simulink model "model_LQR"  (R2022b)
settings: Solver=VariableStepAuto  StartTime=0.0  StopTime=30  RelTol=1e-3
values from neighbouring files (symbols this model uses):
  A_INV = [A_P                                        Z1                  Z3                   B_P ... (first row only)    [model_LQR_code.m]
  A_inv = zeros(15,15)    [model_LQR_code.m]
  B_INV = [Z6 ... (first row only)    [model_LQR_code.m]
  B_inv = zeros(15,4)    [model_LQR_code.m]
  C_f = (0.066*C_b)    (= 0.00220630670953)    [model_LQR_code.m]
  C_INV = [C_inv_w ... (first row only)    [model_LQR_code.m]
  C_inv = zeros(2,15)    [model_LQR_code.m]
  D_INV = zeros(3,2)    [model_LQR_code.m]
  D_inv = zeros(2,4)    [model_LQR_code.m]
  f_b = 50    [model_LQR_code.m]
  G3 = -pinv(G2)    [model_LQR_code.m]
  G33 = -pinv(G22)    [model_LQR_code.m]
  Kic = R_f/ti    (= 1.587)    [model_LQR_code.m]
  Kiv = R_f/tiv    (= 0.1587)    [model_LQR_code.m]
  Kpc = L_f/ti    [model_LQR_code.m]
  Kpv = C_f*wm    [model_LQR_code.m]
  L_f = V_dc/(24*f_sw*delta_IL_max)    [model_LQR_code.m]
  L_g = 1*L_f    [model_LQR_code.m]
  mp = 0.03*50*2*pi/(S_b)    (= 1.88495559215e-06)    [model_LQR_code.m]
  nq = 1*V_m/(S_b)    [model_LQR_code.m]
  R_d = 0.2    [model_LQR_code.m]
  R_f = 0.005*Z_b    (= 0.0004761)    [model_LQR_code.m]
  R_g = 0.005*Z_b    (= 0.0004761)    [model_LQR_code.m]
  S_b = 5e6    (= 5000000)    [model_LQR_code.m]
  T_s = 100e-6    (= 0.0001)    [model_LQR_code.m]
  V_dc = 3*V_m    [model_LQR_code.m]
  V_m = sqrt(2/3)*V_b    [model_LQR_code.m]
  w_b = f_b*2*pi    (= 314.159265359)    [model_LQR_code.m]
  w_c = 0.1*w_b    (= 31.4159265359)    [model_LQR_code.m]
undefined symbols (not defined in the file or in its folder): K, K1
libraries: slpidlib x8, spsabctodq0Lib x6, spsThreePhaseSeriesRLCBranchLib x4, spsPowerdq0InstantaneousLib x3, spsThreePhaseVIMeasurementLib x3, spsdq0toabcLib x3, spsGroundLib x2, spsDCVoltageSourceLib x1, spsPLL3phLib x1, spsPWMGenerator2LevelLib x1, spsPower3phPhasorLib x1, spsThreePhaseProgrammableVoltageSourceLib x1
(part 2 of 2)

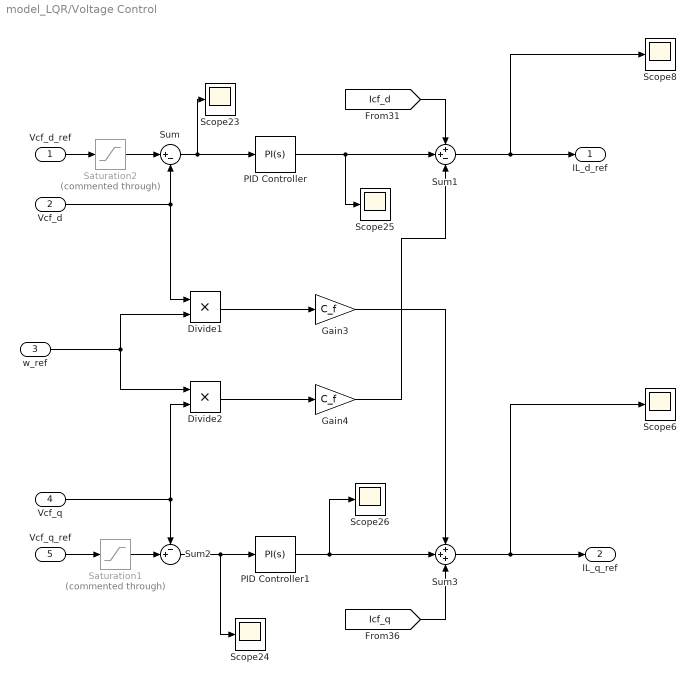
== system model_LQR/Voltage Control ==
  Vcf_d_ref : Inport
  Vcf_d : Inport  Port=2
  w_ref : Inport  Port=3
  Vcf_q : Inport  Port=4
  Vcf_q_ref : Inport  Port=5
  Divide1 : Product  Inputs=**
  Divide2 : Product  Inputs=**
  Gain3 : Gain  Gain=C_f
  Gain4 : Gain  Gain=C_f
  PID Controller : slpidlib/PID Controller  Controller=PI  Form=Parallel  TimeDomain=Continuous-time  UseExternalTs=off  SampleTime=-1  IntegratorMethod=Forward Euler  FilterMethod=Forward Euler  ControllerParametersSource=internal  P=Kpv  I=Kiv  UseKiTs=off  D=0  N=100  UseFilter=on  TunerSelectOption=Transfer Function Based (PID Tuner App)  InitialConditionSource=internal  InitialConditionForIntegrator=0  InitialConditionForFilter=0  DifferentiatorICPrevScaledInput=0  ExternalReset=none  TrackingMode=off  Kt=1  LimitOutput=off  SatLimitsSource=internal  UpperSaturationLimit=75  LowerSaturationLimit=-20  LinearizeAsGain=on  AntiWindupMode=none  Kb=1  LimitIntegrator=off  UpperIntegratorSaturationLimit=inf  LowerIntegratorSaturationLimit=-inf  POutMin=[]  POutMax=[]  IOutMin=[]  IOutMax=[]  DOutMin=[]  DOutMax=[]  NOutMin=[]  NOutMax=[]  SumOutMin=[]  SumOutMax=[]  SaturationOutMin=[]  SaturationOutMax=[]  PParamMin=[]  PParamMax=[]  IParamMin=[]  IParamMax=[]  DParamMin=[]  DParamMax=[]  NParamMin=[]  NParamMax=[]  KbParamMin=[]  KbParamMax=[]  KtParamMin=[]  KtParamMax=[]  KbOutMin=[]  KbOutMax=[]  KtOutMin=[]  KtOutMax=[]  IntegratorOutMin=[]  IntegratorOutMax=[]  FilterOutMin=[]  FilterOutMax=[]  SumI1OutMin=[]  SumI1OutMax=[]  SumI2OutMin=[]  SumI2OutMax=[]  SumI3OutMin=[]  SumI3OutMax=[]  SumI4OutMin=[]  SumI4OutMax=[]  SumDOutMin=[]  SumDOutMax=[]  DifferentiatorOutMin=[]  DifferentiatorOutMax=[]  FilterDiffOutCoefMin=[]  FilterDiffOutCoefMax=[]  ReciprocalOutMin=[]  ReciprocalOutMax=[]  SumDenOutMin=[]  SumDenOutMax=[]  SumNumOutMin=[]  SumNumOutMax=[]  DivideOutMin=[]  DivideOutMax=[]  UdiffTsProdOutMin=[]  UdiffTsProdOutMax=[]  NTsProdOutMin=[]  NTsProdOutMax=[]  UintegralTsProdOutMin=[]  UintegralTsProdOutMax=[]  UngainTsProdOutMin=[]  UngainTsProdOutMax=[]  ClampingZeroOutDataTypeStr=Inherit: Inherit via back propagation  ClampingZeroOutMin=[]  ClampingZeroOutMax=[]  FilterDenConstantOutDataTypeStr=Inherit: Inherit via back propagation  FilterDenConstantOutMin=[]  FilterDenConstantOutMax=[]  PCopyOutDataTypeStr=Inherit: Inherit via back propagation  PCopyOutMin=[]  PCopyOutMax=[]  NCopyOutDataTypeStr=Inherit: Inherit via back propagation  NCopyOutMin=[]  NCopyOutMax=[]  IntegratorContinuousStateAttributes=''  IntegratorStateMustResolveToSignalObject=off  IntegratorRTWStateStorageClass=Auto  FilterContinuousStateAttributes=''  FilterStateMustResolveToSignalObject=off  FilterRTWStateStorageClass=Auto  ParallelPVariant=InternalParameters  IdealPVariant=Disabled  IVariant=InternalParameters  DVariant=Disabled  IntegratorVariant=Continuous  SatVariant=Disabled  AWVariant=Passthrough  PCopyVariant=Disabled  TRVariant=Disabled  FdbkBlocksVariant=Forward  IdealPFdbkVariant=Disabled  SatFdbkVariant=Disabled  DerivativeFilterVariant=Disabled  NVariant=Disabled  NCopyVariant=Disabled_SignalSpec  FilterICVariant=Disabled  IntegratorICVariant=InternalICs  ExternalResetVariant=Disabled  TRSumVariant=Passthrough  SumFdbkVariant=Disabled  SumVariant=Sum_PI  TsampFilterVariant=InternalTs  TsampNgainVariant=Passthrough  TsampIntegralVariant=Passthrough  ExternalSaturationOutDataTypeStr=Inherit: Same as second input
  PID Controller1 : slpidlib/PID Controller  Controller=PI  Form=Parallel  TimeDomain=Continuous-time  UseExternalTs=off  SampleTime=-1  IntegratorMethod=Forward Euler  FilterMethod=Forward Euler  ControllerParametersSource=internal  P=Kpv  I=Kiv  UseKiTs=off  D=0  N=100  UseFilter=on  TunerSelectOption=Transfer Function Based (PID Tuner App)  InitialConditionSource=internal  InitialConditionForIntegrator=0  InitialConditionForFilter=0  DifferentiatorICPrevScaledInput=0  ExternalReset=none  TrackingMode=off  Kt=1  LimitOutput=off  SatLimitsSource=internal  UpperSaturationLimit=250  LowerSaturationLimit=-250  LinearizeAsGain=on  AntiWindupMode=none  Kb=1  LimitIntegrator=off  UpperIntegratorSaturationLimit=inf  LowerIntegratorSaturationLimit=-inf  POutMin=[]  POutMax=[]  IOutMin=[]  IOutMax=[]  DOutMin=[]  DOutMax=[]  NOutMin=[]  NOutMax=[]  SumOutMin=[]  SumOutMax=[]  SaturationOutMin=[]  SaturationOutMax=[]  PParamMin=[]  PParamMax=[]  IParamMin=[]  IParamMax=[]  DParamMin=[]  DParamMax=[]  NParamMin=[]  NParamMax=[]  KbParamMin=[]  KbParamMax=[]  KtParamMin=[]  KtParamMax=[]  KbOutMin=[]  KbOutMax=[]  KtOutMin=[]  KtOutMax=[]  IntegratorOutMin=[]  IntegratorOutMax=[]  FilterOutMin=[]  FilterOutMax=[]  SumI1OutMin=[]  SumI1OutMax=[]  SumI2OutMin=[]  SumI2OutMax=[]  SumI3OutMin=[]  SumI3OutMax=[]  SumI4OutMin=[]  SumI4OutMax=[]  SumDOutMin=[]  SumDOutMax=[]  DifferentiatorOutMin=[]  DifferentiatorOutMax=[]  FilterDiffOutCoefMin=[]  FilterDiffOutCoefMax=[]  ReciprocalOutMin=[]  ReciprocalOutMax=[]  SumDenOutMin=[]  SumDenOutMax=[]  SumNumOutMin=[]  SumNumOutMax=[]  DivideOutMin=[]  DivideOutMax=[]  UdiffTsProdOutMin=[]  UdiffTsProdOutMax=[]  NTsProdOutMin=[]  NTsProdOutMax=[]  UintegralTsProdOutMin=[]  UintegralTsProdOutMax=[]  UngainTsProdOutMin=[]  UngainTsProdOutMax=[]  ClampingZeroOutDataTypeStr=Inherit: Inherit via back propagation  ClampingZeroOutMin=[]  ClampingZeroOutMax=[]  FilterDenConstantOutDataTypeStr=Inherit: Inherit via back propagation  FilterDenConstantOutMin=[]  FilterDenConstantOutMax=[]  PCopyOutDataTypeStr=Inherit: Inherit via back propagation  PCopyOutMin=[]  PCopyOutMax=[]  NCopyOutDataTypeStr=Inherit: Inherit via back propagation  NCopyOutMin=[]  NCopyOutMax=[]  IntegratorContinuousStateAttributes=''  IntegratorStateMustResolveToSignalObject=off  IntegratorRTWStateStorageClass=Auto  FilterContinuousStateAttributes=''  FilterStateMustResolveToSignalObject=off  FilterRTWStateStorageClass=Auto  ParallelPVariant=InternalParameters  IdealPVariant=Disabled  IVariant=InternalParameters  DVariant=Disabled  IntegratorVariant=Continuous  SatVariant=Disabled  AWVariant=Passthrough  PCopyVariant=Disabled  TRVariant=Disabled  FdbkBlocksVariant=Forward  IdealPFdbkVariant=Disabled  SatFdbkVariant=Disabled  DerivativeFilterVariant=Disabled  NVariant=Disabled  NCopyVariant=Disabled_SignalSpec  FilterICVariant=Disabled  IntegratorICVariant=InternalICs  ExternalResetVariant=Disabled  TRSumVariant=Passthrough  SumFdbkVariant=Disabled  SumVariant=Sum_PI  TsampFilterVariant=InternalTs  TsampNgainVariant=Passthrough  TsampIntegralVariant=Passthrough  ExternalSaturationOutDataTypeStr=Inherit: Same as second input
  Saturation1 : Saturate  Commented=through  UpperLimit=30  LowerLimit=-10
  Saturation2 : Saturate  Commented=through  UpperLimit=1.4*V_m  LowerLimit=0.75*V_m
  Scope{6,8,23..26} (6 alike) : Scope
  Sum : Sum  Inputs=|+-
  Sum1 : Sum  Inputs=++-
  Sum2 : Sum  Inputs=-+|
  Sum3 : Sum  Inputs=+++
  IL_d_ref : Outport
  IL_q_ref : Outport  Port=2
  wires:
  Sum/1 -> Scope23/1, PID Controller/1
  PID Controller/1 -> Scope25/1, Sum1/2
  PID Controller1/1 -> Scope26/1, Sum3/2
  [Icf_q] -> Sum3/3
  Gain3/1 -> Sum3/1
  Sum2/1 -> Scope24/1, PID Controller1/1
  [Icf_d] -> Sum1/1
  Divide1/1 -> Gain3/1
  Sum3/1 -> IL_q_ref/1, Scope6/1
  Sum1/1 -> IL_d_ref/1, Scope8/1
  Divide2/1 -> Gain4/1
  Gain4/1 -> Sum1/3
  Vcf_d_ref/1 -> Saturation2/1
  Vcf_d/1 -> Divide1/1, Sum/2
  w_ref/1 -> Divide2/1, Divide1/2
  Vcf_q_ref/1 -> Saturation1/1
  Vcf_q/1 -> Divide2/2, Sum2/1
  Saturation1/1 -> Sum2/2
  Saturation2/1 -> Sum/1

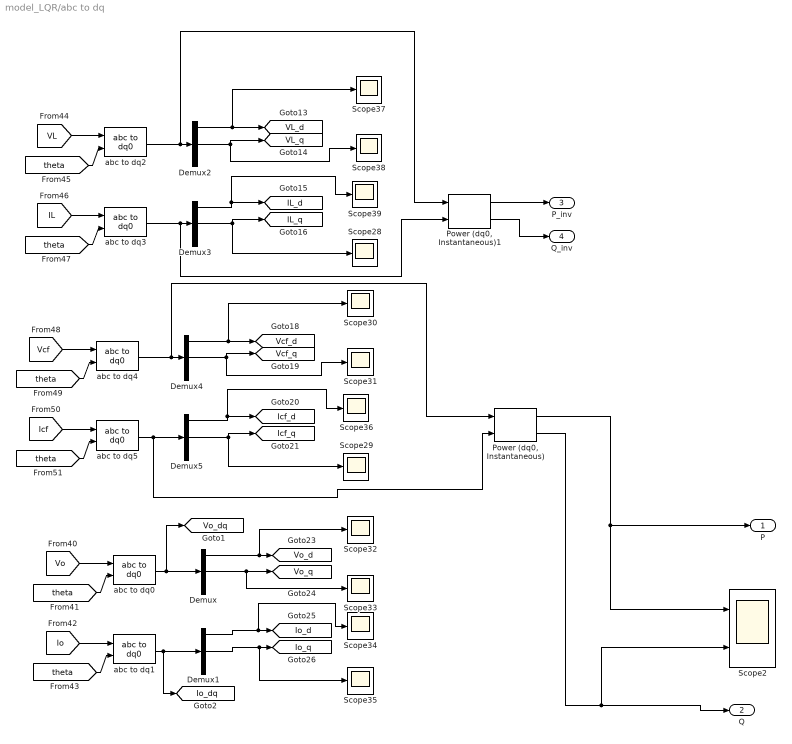
== system model_LQR/abc to dq ==
  Demux{,1..5} (6 alike) : Demux  Outputs=3
  "Power (dq0, Instantaneous)" : spsPowerdq0InstantaneousLib/Power (dq0, Instantaneous)
      settings: LibrarySourceBlock=|
      | sps_lib/Sensors and Measurements/Power
      | (dq0, Instantaneous)
  "Power (dq0, Instantaneous)1" : spsPowerdq0InstantaneousLib/Power (dq0, Instantaneous)
      settings: LibrarySourceBlock=|
      | sps_lib/Sensors and Measurements/Power
      | (dq0, Instantaneous)
  Scope2 : Scope  NumInputPorts=2
  Scope{28..39} (12 alike) : Scope
  abc to dq{0..5} (6 alike) : spsabctodq0Lib/abc to dq0  Alignment=90 degrees behind phase A axis
  P : Outport
  Q : Outport  Port=2
  P_inv : Outport  Port=3
  Q_inv : Outport  Port=4
  tag scope: IL_d=global, IL_q=global, Icf_d=global, Icf_q=global, Io_d=global, Io_dq=global, Io_q=global, VL_d=global, VL_q=global, Vcf_d=global, Vcf_q=global, Vo_d=global, Vo_dq=global, Vo_q=global
  wires:
  [IL] -> abc to dq3/1
  Demux2/1 -> Scope37/1, [VL_d]
  abc to dq4/1 -> "Power (dq0, Instantaneous)"/1, Demux4/1
  Demux1/1 -> Scope34/1, [Io_d]
  abc to dq1/1 -> [Io_dq], Demux1/1
  Demux5/1 -> Scope36/1, [Icf_d]
  Demux2/2 -> Scope38/1, [VL_q]
  abc to dq0/1 -> [Vo_dq], Demux/1
  Demux/2 -> Scope33/1, [Vo_q]
  "Power (dq0, Instantaneous)"/1 -> Scope2/1, P/1
  Demux4/1 -> Scope30/1, [Vcf_d]
  Demux/1 -> Scope32/1, [Vo_d]
  "Power (dq0, Instantaneous)"/2 -> Scope2/2, Q/1
  [theta] -> abc to dq2/2
  [theta] -> abc to dq3/2
  [VL] -> abc to dq2/1
  [Vcf] -> abc to dq4/1
  abc to dq5/1 -> "Power (dq0, Instantaneous)"/2, Demux5/1
  [theta] -> abc to dq4/2
  Demux4/2 -> Scope31/1, [Vcf_q]
  [theta] -> abc to dq0/2
  Demux3/2 -> Scope28/1, [IL_q]
  Demux3/1 -> Scope39/1, [IL_d]
  abc to dq3/1 -> "Power (dq0, Instantaneous)1"/2, Demux3/1
  Demux1/2 -> Scope35/1, [Io_q]
  [theta] -> abc to dq1/2
  abc to dq2/1 -> "Power (dq0, Instantaneous)1"/1, Demux2/1
  Demux5/2 -> Scope29/1, [Icf_q]
  [theta] -> abc to dq5/2
  [Icf] -> abc to dq5/1
  [Io] -> abc to dq1/1
  [Vo] -> abc to dq0/1
  "Power (dq0, Instantaneous)1"/1 -> P_inv/1
  "Power (dq0, Instantaneous)1"/2 -> Q_inv/1

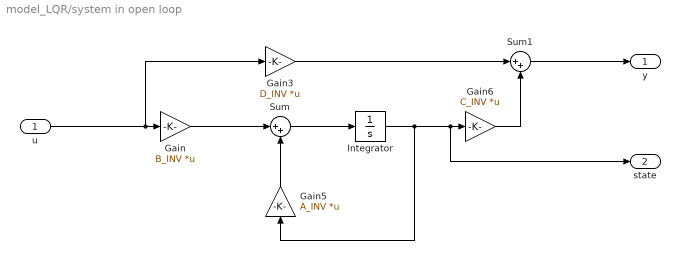
== system model_LQR/system in open loop ==
  u : Inport
  Gain : Gain  Gain=B_INV  Multiplication=Matrix(K*u)
  Gain3 : Gain  Gain=D_INV  Multiplication=Matrix(K*u)
  Gain5 : Gain  Gain=A_INV  Multiplication=Matrix(K*u)
  Gain6 : Gain  Gain=C_INV  Multiplication=Matrix(K*u)
  Integrator : Integrator
  Sum : Sum  Inputs=|++
  Sum1 : Sum  Inputs=|++
  y : Outport
  state : Outport  Port=2
  wires:
  Gain3/1 -> Sum1/1
  u/1 -> Gain3/1, Gain/1
  Gain/1 -> Sum/1
  Gain6/1 -> Sum1/2
  Integrator/1 -> Gain5/1, state/1, Gain6/1
  Gain5/1 -> Sum/2
  Sum/1 -> Integrator/1
  Sum1/1 -> y/1

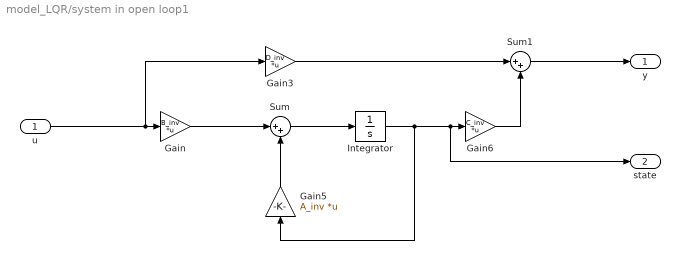
== system model_LQR/system in open loop1 ==
  u : Inport
  Gain : Gain  Gain=B_inv  Multiplication=Matrix(K*u)
  Gain3 : Gain  Gain=D_inv  Multiplication=Matrix(K*u)
  Gain5 : Gain  Gain=A_inv  Multiplication=Matrix(K*u)
  Gain6 : Gain  Gain=C_inv  Multiplication=Matrix(K*u)
  Integrator : Integrator
  Sum : Sum  Inputs=|++
  Sum1 : Sum  Inputs=|++
  y : Outport
  state : Outport  Port=2
  wires:
  Gain3/1 -> Sum1/1
  u/1 -> Gain3/1, Gain/1
  Gain/1 -> Sum/1
  Gain6/1 -> Sum1/2
  Integrator/1 -> Gain5/1, state/1, Gain6/1
  Gain5/1 -> Sum/2
  Sum/1 -> Integrator/1
  Sum1/1 -> y/1
